simulink model "Properties_PID_Controller_without_RL"  (R2015a)
settings: Solver=FixedStepDiscrete  StartTime=0.0  StopTime=10.0  FixedStep=delta_t  RelTol=1e-3
undefined symbols (not defined in the file): delta_t, psi_dot_max, psi_max
settings Model: Creator=Kerianne  LastModifiedBy=Kerianne
settings DataIOCC: SaveFormat=Structure
settings OptimizationCC: InlineParams=on  ExpressionDepthLimit=2147483647
settings DebuggingCC: UnderspecifiedInitializationDetection=Classic  MergeDetectMultiDrivingBlocksExec=none  SolverPrmCheckMsg=warning  StateNameClashWarn=warning

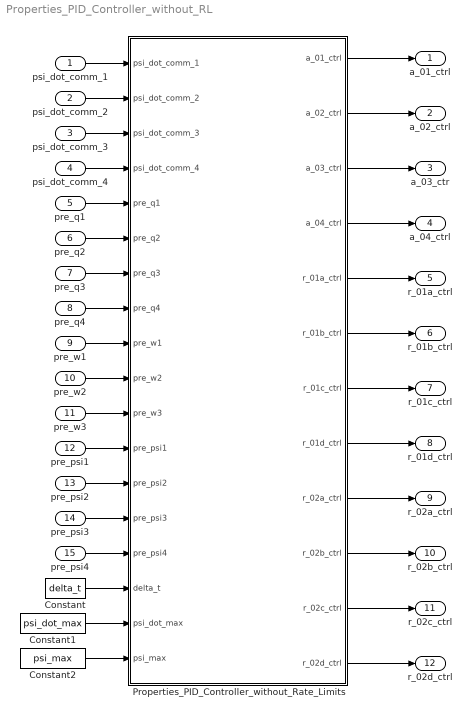
== system Properties_PID_Controller_without_RL ==
  psi_dot_comm_1 : Inport
  psi_dot_comm_2 : Inport  Port=2
  "psi_dot_comm_3 " : Inport  Port=3
  psi_dot_comm_4 : Inport  Port=4
  pre_q1 : Inport  Port=5
  pre_q2 : Inport  Port=6
  pre_q3 : Inport  Port=7
  pre_q4 : Inport  Port=8
  pre_w1 : Inport  Port=9
  pre_w2 : Inport  Port=10
  pre_w3 : Inport  Port=11
  pre_psi1 : Inport  Port=12
  pre_psi2 : Inport  Port=13
  pre_psi3 : Inport  Port=14
  pre_psi4 : Inport  Port=15
  Constant : Constant  Value=delta_t
  Constant1 : Constant  Value=psi_dot_max
  Constant2 : Constant  Value=psi_max
  Properties_PID_Controller_without_Rate_Limits : MATLAB Function  TreatAsAtomicUnit=on
  a_01_ctrl : Outport  OutDataTypeStr=boolean
  a_02_ctrl : Outport  Port=2  OutDataTypeStr=boolean
  a_03_ctr : Outport  Port=3  OutDataTypeStr=boolean
  a_04_ctrl : Outport  Port=4  OutDataTypeStr=boolean
  "r_01a_ctrl " : Outport  Port=5  OutDataTypeStr=boolean
  r_01b_ctrl : Outport  Port=6  OutDataTypeStr=boolean
  r_01c_ctrl : Outport  Port=7  OutDataTypeStr=boolean
  r_01d_ctrl : Outport  Port=8  OutDataTypeStr=boolean
  r_02a_ctrl : Outport  Port=9  OutDataTypeStr=boolean
  r_02b_ctrl : Outport  Port=10  OutDataTypeStr=boolean
  r_02c_ctrl : Outport  Port=11  OutDataTypeStr=boolean
  r_02d_ctrl : Outport  Port=12  OutDataTypeStr=boolean
  wires:
  Properties_PID_Controller_without_Rate_Limits/12(r_02d_ctrl) -> r_02d_ctrl/1
  Properties_PID_Controller_without_Rate_Limits/11(r_02c_ctrl) -> r_02c_ctrl/1
  Properties_PID_Controller_without_Rate_Limits/10(r_02b_ctrl) -> r_02b_ctrl/1
  Properties_PID_Controller_without_Rate_Limits/9(r_02a_ctrl) -> r_02a_ctrl/1
  Properties_PID_Controller_without_Rate_Limits/1(a_01_ctrl) -> a_01_ctrl/1
  Properties_PID_Controller_without_Rate_Limits/7(r_01c_ctrl) -> r_01c_ctrl/1
  Properties_PID_Controller_without_Rate_Limits/6(r_01b_ctrl) -> r_01b_ctrl/1
  Properties_PID_Controller_without_Rate_Limits/8(r_01d_ctrl) -> r_01d_ctrl/1
  psi_dot_comm_1/1 -> Properties_PID_Controller_without_Rate_Limits/1(psi_dot_comm_1)
  psi_dot_comm_2/1 -> Properties_PID_Controller_without_Rate_Limits/2(psi_dot_comm_2)
  "psi_dot_comm_3 "/1 -> Properties_PID_Controller_without_Rate_Limits/3(psi_dot_comm_3)
  psi_dot_comm_4/1 -> Properties_PID_Controller_without_Rate_Limits/4(psi_dot_comm_4)
  Constant/1 -> Properties_PID_Controller_without_Rate_Limits/16(delta_t)
  Constant2/1 -> Properties_PID_Controller_without_Rate_Limits/18(psi_max)
  Constant1/1 -> Properties_PID_Controller_without_Rate_Limits/17(psi_dot_max)
  pre_q1/1 -> Properties_PID_Controller_without_Rate_Limits/5(pre_q1)
  pre_q3/1 -> Properties_PID_Controller_without_Rate_Limits/7(pre_q3)
  pre_q2/1 -> Properties_PID_Controller_without_Rate_Limits/6(pre_q2)
  pre_q4/1 -> Properties_PID_Controller_without_Rate_Limits/8(pre_q4)
  pre_psi4/1 -> Properties_PID_Controller_without_Rate_Limits/15(pre_psi4)
  pre_psi3/1 -> Properties_PID_Controller_without_Rate_Limits/14(pre_psi3)
  pre_psi2/1 -> Properties_PID_Controller_without_Rate_Limits/13(pre_psi2)
  pre_psi1/1 -> Properties_PID_Controller_without_Rate_Limits/12(pre_psi1)
  pre_w3/1 -> Properties_PID_Controller_without_Rate_Limits/11(pre_w3)
  pre_w2/1 -> Properties_PID_Controller_without_Rate_Limits/10(pre_w2)
  pre_w1/1 -> Properties_PID_Controller_without_Rate_Limits/9(pre_w1)
  Properties_PID_Controller_without_Rate_Limits/5(r_01a_ctrl) -> "r_01a_ctrl "/1
  Properties_PID_Controller_without_Rate_Limits/4(a_04_ctrl) -> a_04_ctrl/1
  Properties_PID_Controller_without_Rate_Limits/3(a_03_ctrl) -> a_03_ctr/1
  Properties_PID_Controller_without_Rate_Limits/2(a_02_ctrl) -> a_02_ctrl/1

== matlab function Properties_PID_Controller_without_RL/Properties_PID_Controller_without_Rate_Limits ==
  data: psi_dot_comm_1 input; a_01_ctrl output; a_02_ctrl output; a_03_ctrl output; a_04_ctrl output; r_01a_ctrl output; r_01b_ctrl output; r_01c_ctrl output; r_01d_ctrl output; r_02a_ctrl output; r_02b_ctrl output; r_02c_ctrl output; r_02d_ctrl output; psi_dot_comm_2 input; psi_dot_comm_3 input; psi_dot_comm_4 input; pre_q1 input; pre_q2 input; pre_q3 input; pre_q4 input; pre_w1 input; pre_w2 input; pre_w3 input; pre_psi1 input; pre_psi2 input; pre_psi3 input; pre_psi4 input; delta_t input; psi_dot_max input; psi_max input
function [a_01_ctrl,a_02_ctrl,a_03_ctrl,a_04_ctrl,r_01a_ctrl,r_01b_ctrl,r_01c_ctrl,r_01d_ctrl,r_02a_ctrl,r_02b_ctrl,r_02c_ctrl,r_02d_ctrl] = verification_condition(psi_dot_comm_1,psi_dot_comm_2,psi_dot_comm_3,psi_dot_comm_4,pre_q1,pre_q2,pre_q3,pre_q4,pre_w1,pre_w2,pre_w3,pre_psi1,pre_psi2,pre_psi3,pre_psi4,delta_t,psi_dot_max,psi_max)
% Properties for Reaction Wheel Control
% Author: Kerianne Gross, AFRL/RQQA, kerianne.gross@us.af.mil
% Last Updated: 20 November 2015 

MAX_PSI_DOT_RW = psi_dot_max;
MAX_PSI_RW = psi_max; 

%% Assumptions
a_01_ctrl = pre_psi1 <= MAX_PSI_RW && pre_psi1 >= -MAX_PSI_RW;
a_02_ctrl = pre_psi2 <= MAX_PSI_RW && pre_psi2 >= -MAX_PSI_RW;
a_03_ctrl = pre_psi3 <= MAX_PSI_RW && pre_psi3 >= -MAX_PSI_RW;
a_04_ctrl = pre_psi4 <= MAX_PSI_RW && pre_psi4 >= -MAX_PSI_RW;

%% Guarantees (Proof Objectives)
%R01 The commanded change of angular velocity from the control 
%    algorithm shall not exceed the maximum allowable angular acceleration
%    of the reaction wheel.
r_01a_ctrl = (psi_dot_comm_1 <= MAX_PSI_DOT_RW) && (psi_dot_comm_1 >= -MAX_PSI_DOT_RW); %[rad_p_s_2]
r_01b_ctrl = (psi_dot_comm_2 <= MAX_PSI_DOT_RW) && (psi_dot_comm_2 >= -MAX_PSI_DOT_RW); %[rad_p_s_2]
r_01c_ctrl = (psi_dot_comm_3 <= MAX_PSI_DOT_RW) && (psi_dot_comm_3 >= -MAX_PSI_DOT_RW); %[rad_p_s_2]
r_01d_ctrl = (psi_dot_comm_4 <= MAX_PSI_DOT_RW) && (psi_dot_comm_4 >= -MAX_PSI_DOT_RW); %[rad_p_s_2]
%R02 The control algorithm prediction of reaction wheel angular velocity as a result of the commanded change of 
%    angular velocity shall not exceed the maximum allowable angular velocity of the reaction wheel.
r_02a_ctrl = (pre_psi1 + psi_dot_comm_1*(delta_t) <= MAX_PSI_RW) && (pre_psi1 + psi_dot_comm_1*(delta_t) >= -MAX_PSI_RW);  
r_02b_ctrl = (pre_psi2 + psi_dot_comm_2*(delta_t) <= MAX_PSI_RW) && (pre_psi2 + psi_dot_comm_2*(delta_t) >= -MAX_PSI_RW);  
r_02c_ctrl = (pre_psi3 + psi_dot_comm_3*(delta_t) <= MAX_PSI_RW) && (pre_psi3 + psi_dot_comm_3*(delta_t) >= -MAX_PSI_RW);  
r_02d_ctrl = (pre_psi4 + psi_dot_comm_4*(delta_t) <= MAX_PSI_RW) && (pre_psi4 + psi_dot_comm_4*(delta_t) >= -MAX_PSI_RW);
